simulink library "dspddes2"  (Simulink 3.00)
values from neighbouring files (symbols this model uses):
  a = []    [dspfdes.m]    (also in dsprprim.m = a-Mi)
  b = []    [dspfdes.m]    (also in dsprprim.m = b+Li)
  c = []    [dspfdes.m]    (also in liblinks.m = cell2struct(v,f,1); sbufscop.m = 'auto')
  d = []    [dspfdes.m]    (also in dsprprim.m = ['x[' num2str(Mi) 'n/' num2str(Li) ']']; resave_mdl.m = dir('*.mdl'); sbufscop.m = abs(magMax-magMin); sdspfscope.m = get(block_data.hframenum(2),'userdata'))
libraries: dsparch2 x6
settings Model: Creator=dshpak  LastModifiedBy=thartley

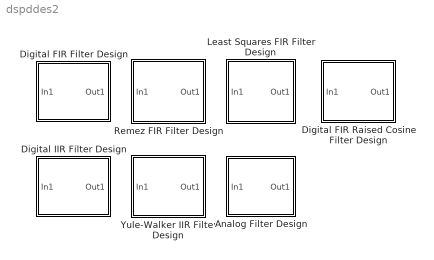
== system dspddes2 ==
  Analog Filter Design : Subsystem  mask(Analog Filter Design){method=Butterworth, filttype=Lowpass, N=8, Wlo=30, Whi=80, Rp=2, Rs=40}
      mask prompts: method "Design method:"; filttype "Filter type:"; N "Filter order:"; Wlo "Passband edge frequency (rads/sec):"; Whi "Should not be visible!"; Rp "Passband ripple in dB:"; Rs "Stopband attenuation in dB:"
      mask help: Design one of several standard analog filters, implemented in state-space form.
      mask init:
      | [a,b,c,d,h,w,str]=dspblkanalog('design', method,filttype,N,Wlo,Whi,Rp,Rs);
      mask Help: web(dspbhelp);
      mask StyleString: popup(Butterworth|Chebyshev I|Chebyshev II|Elliptic),popup(Lowpass|Highpass|Bandpass|Bandstop),edit,edit,edit,edit,edit
      mask CallbackString: dspblkanalog|dspblkanalog|||||
      mask Display: plot(w,h); text(.05,.9,str);
  Digital FIR Filter Design : Subsystem  mask(Digital FIR Filter Design){filttype=Lowpass, N=22, Wlo=0.4, Whi=0.6, W0=[.2 .5 .8], g0=1, W1=[0 .2 .3 .6 .8 1], gains=[1 .5 0 0 1 .5], wintype=Hamming, Rs=10, Kbeta=5, frame=off, numChans=1}
      mask prompts: filttype "Filter type:"; N "Filter order:"; Wlo "Cutoff frequency (0 to 1):"; Whi "Upper cutoff frequency:"; W0 "Cutoff frequency vector (0 < f < 1):"; g0 "Gain in the first band:"; W1 "Frequency vector (including 0 and 1):"; gains "Gains at these frequencies:"; wintype "Window type:"; Rs "Stopband attenuation in dB:"; Kbeta "Beta:"; frame "Frame-based inputs"; numChans "Number of channels:"
      mask help: Implements various window-based FIR filter designs using the Signal Processing Toolbox's "fir1" and "fir2" filter design commands. The gain at each "cutoff frequency" is the average of the gains in the adjacent bands (usually 0.5).
      mask init:
      | [b,h,w,str]=dspblkfir('design',filttype,N,Wlo,Whi,W0,g0,W1,gains,wintype,Rs, Kbeta);
      | numChans = dspblkfir('update', numChans);
      mask Help: web(dspbhelp);
      mask StyleString: popup(Lowpass|Highpass|Bandpass|Bandstop|Multiband|Arbitrary Shape (fir2)),edit,edit,edit,edit,popup(0|1),edit,edit,popup(Bartlett|Blackman|Boxcar|Chebyshev|Hamming|Hann|Hanning|Kaiser|Triangular),edit,edit,checkbox,edit
      mask CallbackString: dspblkfir||||||||dspblkfir|||dspblkfir|
      mask Display: plot(w,h); text(.05,.9,str);
  Digital FIR Raised Cosine Filter Design : Subsystem  mask(Digital FIR Raised Cosine Filter Design){filter_order=63, upper_cutoff_freq=0.5, enable_sqrt_design=on, rolloff_type=Rolloff factor, transition_bw=0.4, rolloff_factor=0.6, window_type=Boxcar, Rs=5, Kbeta=10, InitCond=0, frame_based=off, num_chans=1}
      mask prompts: filter_order "Filter order:"; upper_cutoff_freq "Upper cutoff frequency (0 to 1):"; enable_sqrt_design "Square-root raised cosine filter"; rolloff_type "Design method:"; transition_bw "Transition bandwidth (0 < Df < 1):"; rolloff_factor "Rolloff factor (0 to 1):"; window_type "Window type:"; Rs "Stopband attenuation in dB:"; Kbeta "Beta:"; InitCond "Initial conditions:"; frame_based "Frame-based inputs"; num_chans "Number of channels:"
      mask help: Linear phase digital FIR lowpass raised cosine filter.
      mask init:
      | [str,h,w,b]= dspblkfirrcos('design',filter_order,upper_cutoff_freq,rolloff_type,transition_bw,rolloff_factor, window_type, Rs, enable_sqrt_design, frame_based,num_chans, Kbeta);
      | dspblkfirrcos('update');
      mask Help: web(dspbhelp);
      mask StyleString: edit,edit,checkbox,popup(Transition bandwidth|Rolloff factor),edit,edit,popup(Bartlett|Blackman|Boxcar|Chebyshev|Hamming|Hann|Hanning|Kaiser|Triangular),edit,edit,edit,checkbox,edit
      mask CallbackString: |||dspblkfirrcos|||dspblkfirrcos||||dspblkfirrcos|
      mask Display:
      | plot(w,h);
      | text(.05,.9,str);
  Digital IIR Filter Design : Subsystem  mask(Digital IIR Filter Design){method=Butterworth, filttype=Lowpass, N=4, Wlo=0.4, Whi=0.6, Rp=2, Rs=20, frame=off, numCHANS=1}
      mask prompts: method "Design method:"; filttype "Filter type:"; N "Filter order:"; Wlo "Lower passband edge frequency (0 to 1):"; Whi "Upper passband edge frequency:"; Rp "Passband ripple in dB:"; Rs "Stopband attenuation in dB:"; frame "Frame-based inputs"; numCHANS "Number of channels:"
      mask help: Design one of several standard IIR filters, implemented in direct form.
      mask init:
      | [b,a,h,w,str] = dspblkiir('design',method,filttype,N,...
      |                                               Wlo,Whi,Rp,Rs);
      | numCHANS = dspblkiir('update',  numCHANS);
      mask Help: web(dspbhelp);
      mask StyleString: popup(Butterworth|Chebyshev I|Chebyshev II|Elliptic),popup(Lowpass|Highpass|Bandpass|Bandstop),edit,edit,edit,edit,edit,checkbox,edit
      mask CallbackString: dspblkiir|dspblkiir||||||dspblkiir|
      mask Display: plot(w,h); text(.05,.9,str);
  Least Squares FIR Filter Design : Subsystem  mask(Least Squares FIR Filter Design){filttype=Multiband, N=12, F=[0 0.3 0.6 1], A=[0 0 1 1], W=[1 1], frame=off, numChans=1}
      mask prompts: filttype "Filter type:"; N "Filter order:"; F "Band-edge frequency vector (including 0 and 1):"; A "Gains at these frequencies:"; W "Weights (one per band):"; frame "Frame-based inputs"; numChans "Number of channels:"
      mask help: Least-squares linear phase FIR filter.
      mask init:
      | [b,h,w,str] = dspblkfirls('design',filttype,N,F,A,W);
      | numChans = dspblkfirls('update', numChans);
      mask Help: web(dspbhelp);
      mask StyleString: popup(Multiband|Hilbert Transformer|Differentiator),edit,edit,edit,edit,checkbox,edit
      mask CallbackString: |||||dspblkfirls|
      mask Display: plot(w,h); text(.05,.9,str);
  Remez FIR Filter Design : Subsystem  mask(Remez FIR Filter Design){filttype=Multiband, F=[0 0.4 0.5 1], A=[1 1 0 0], W=[1 1], N=23, frame=off, numCHANS=1}
      mask prompts: filttype "Filter type:"; F "Band-edge frequency vector (including 0 and 1):"; A "Gains at these frequencies:"; W "Weights (one per band):"; N "Filter order:"; frame "Frame-based inputs"; numCHANS "Number of channels:"
      mask help: Parks-McClellan linear phase FIR filter.
      mask init:
      | [b,h,w,str] = dspblkremez('design', filttype,N,F,A,W);
      | numCHANS = dspblkremez('update', numCHANS);
      mask Help: web(dspbhelp);
      mask StyleString: popup(Multiband|Hilbert Transformer|Differentiator),edit,edit,edit,edit,checkbox,edit
      mask CallbackString: |||||dspblkremez|
      mask Display: plot(w,h); text(.05,.9,str);
  Yule-Walker IIR Filter Design : Subsystem  mask(Yule-Walker IIR Filter Design){N=8, F=[0 .4 .6 1], A=[1 1 0 0], frame=off, numCHANS=1}
      mask prompts: N "Filter order:"; F "Band-edge frequency vector (including 0 and 1):"; A "Magnitudes at these frequencies:"; frame "Frame-based inputs"; numCHANS "Number of channels:"
      mask help: Yule-Walker IIR filter design.
      mask init:
      | [b,a,h,w,str] = dspblkyule('design', N,F,A);
      | numCHANS = dspblkyule('update', numCHANS);
      mask Help: web(dspbhelp);
      mask CallbackString: |||dspblkyule|
      mask Display: plot(w,h); text(.05,.9,str);

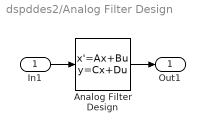
== system dspddes2/Analog Filter Design ==
  In1 : Inport  Port=1  PortWidth=-1  SampleTime=-1  DataType=auto
      settings: SignalType=auto
  Analog Filter Design : StateSpace  A=a  B=b  C=c  D=d  X0=0
  Out1 : Outport  Port=1  InitialOutput=0
  wires:
  In1/1 -> Analog Filter Design/1
  Analog Filter Design/1 -> Out1/1

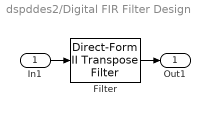
== system dspddes2/Digital FIR Filter Design ==
  In1 : Inport  Port=1  PortWidth=-1  SampleTime=-1  DataType=auto
      settings: SignalType=auto
  Filter : dsparch2/Direct-Form II Transpose Filter  num=b  den=1  ic=0  frame=off  numCHANS=numChans
  Out1 : Outport  Port=1  InitialOutput=0
  wires:
  In1/1 -> Filter/1
  Filter/1 -> Out1/1

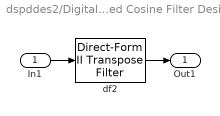
== system dspddes2/Digital FIR Raised Cosine Filter Design ==
  In1 : Inport  Port=1  PortWidth=-1  SampleTime=-1  DataType=auto
      settings: SignalType=auto
  df2 : dsparch2/Direct-Form II Transpose Filter  num=b  den=1  ic=InitCond  frame=off  numCHANS=num_chans
  Out1 : Outport  Port=1
  wires:
  In1/1 -> df2/1
  df2/1 -> Out1/1

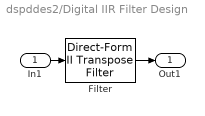
== system dspddes2/Digital IIR Filter Design ==
  In1 : Inport  Port=1  PortWidth=-1  SampleTime=-1  DataType=auto
      settings: SignalType=auto
  Filter : dsparch2/Direct-Form II Transpose Filter  num=b  den=a  ic=0  frame=off  numCHANS=numCHANS
  Out1 : Outport  Port=1  InitialOutput=0
  wires:
  In1/1 -> Filter/1
  Filter/1 -> Out1/1

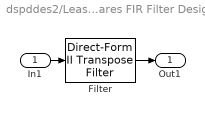
== system dspddes2/Least Squares FIR Filter Design ==
  In1 : Inport  Port=1  PortWidth=-1  SampleTime=-1  DataType=auto
      settings: SignalType=auto
  Filter : dsparch2/Direct-Form II Transpose Filter  num=b  den=1  ic=0  frame=off  numCHANS=numChans
  Out1 : Outport  Port=1  InitialOutput=0
  wires:
  In1/1 -> Filter/1
  Filter/1 -> Out1/1

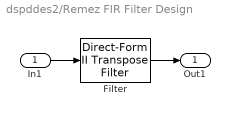
== system dspddes2/Remez FIR Filter Design ==
  In1 : Inport  Port=1  PortWidth=-1  SampleTime=-1  DataType=auto
      settings: SignalType=auto
  Filter : dsparch2/Direct-Form II Transpose Filter  num=b  den=1  ic=0  frame=off  numCHANS=numCHANS
  Out1 : Outport  Port=1  InitialOutput=0
  wires:
  Filter/1 -> Out1/1
  In1/1 -> Filter/1

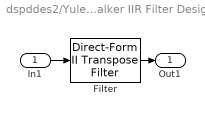
== system dspddes2/Yule-Walker IIR Filter Design ==
  In1 : Inport  Port=1  PortWidth=-1  SampleTime=-1  DataType=auto
      settings: SignalType=auto
  Filter : dsparch2/Direct-Form II Transpose Filter  num=b  den=a  ic=0  frame=off  numCHANS=numCHANS
  Out1 : Outport  Port=1  InitialOutput=0
  wires:
  In1/1 -> Filter/1
  Filter/1 -> Out1/1
